simulink model "modmbkkv"  (Simulink 7.7)
settings: Solver=ode45  StartTime=0.0  StopTime=10.0  RelTol=1e-3
settings Model: Creator=Stijn  LastModifiedBy=Stijn
settings DebuggingCC: SolverPrmCheckMsg=none

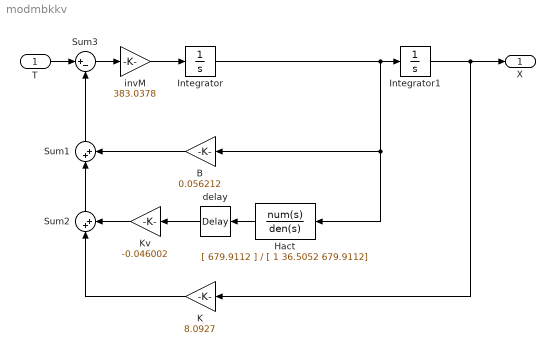
== system modmbkkv ==
  T : Inport
  B : Gain  Gain=0.056212
  Hact : TransferFcn  Numerator=[ 679.9112 ]  Denominator=[ 1 36.5052 679.9112]
  Integrator : Integrator
  Integrator1 : Integrator
  K : Gain  Gain=8.0927
  Kv : Gain  Gain=-0.046002
  Sum1 : Sum  Inputs=|++
  Sum2 : Sum  Inputs=|++
  Sum3 : Sum  Inputs=|+-
  delay : TransportDelay  DelayTime=0.048172
  invM : Gain  Gain=383.0378
  X : Outport
  wires:
  T/1 -> Sum3/1
  Sum3/1 -> invM/1
  invM/1 -> Integrator/1
  Integrator/1 -> Integrator1/1, B/1, Hact/1
  Integrator1/1 -> X/1, K/1
  Hact/1 -> delay/1
  delay/1 -> Kv/1
  B/1 -> Sum1/2
  Sum1/1 -> Sum3/2
  Sum2/1 -> Sum1/1
  K/1 -> Sum2/1
  Kv/1 -> Sum2/2
